simulink model "GFL_inverter"  (R2025a)
settings: Solver=ode4  StartTime=0.0  StopTime=8.5  FixedStep=1e-6  RelTol=1e-3
values from neighbouring files (symbols this model uses):
  An1 = amp1*funn    [dq_saopin_for_GFL_inverter.m]
  An2 = 0    [dq_saopin_for_GFL_inverter.m]
  An3 = 0    [dq_saopin_for_GFL_inverter.m]
  An4 = 0    [dq_saopin_for_GFL_inverter.m]
  An5 = 0    [dq_saopin_for_GFL_inverter.m]
  Ap1 = amp1*funp    [dq_saopin_for_GFL_inverter.m]
  Ap2 = 0    [dq_saopin_for_GFL_inverter.m]
  Ap3 = 0    [dq_saopin_for_GFL_inverter.m]
  Ap4 = 0    [dq_saopin_for_GFL_inverter.m]
  Ap5 = 0    [dq_saopin_for_GFL_inverter.m]
  hp1 = f    [dq_saopin_for_GFL_inverter.m]
  hp2 = f    [dq_saopin_for_GFL_inverter.m]
  hp3 = f    [dq_saopin_for_GFL_inverter.m]
  hp4 = f    [dq_saopin_for_GFL_inverter.m]
  hp5 = f    [dq_saopin_for_GFL_inverter.m]
  t_inj = 7.5    [dq_saopin_for_GFL_inverter.m]
  Ts = 5e-6    (= 5e-06)    [dq_saopin_for_GFL_inverter.m]
undefined symbols (not defined in the file or in its folder): DiscIntNeverNeededParam, level
libraries: powerlib_extras x37, spsControlledVoltageSourceLib x18, spsThreePhaseVIMeasurementLib x7, slpidlib x4, simulink_extras x4, spsabctodq0Lib x3, spsSeriesRLCBranchLib x2, spsUniversalBridgeLib x2, spsMultimeterLib x2, spsThreePhaseProgrammableVoltageSourceLib x1, spsGroundLib x1, spsIGBTDiodeLib x1
(part 1 of 2)
settings Model: SimulationMode=accelerator  Creator=18829  LastModifiedBy=wz
settings SolverCC: AlgebraicLoopSolver=TrustRegion
settings DataIOCC: ReturnWorkspaceOutputs=off
settings OptimizationCC: ReuseModelBlockBuffer=off
settings DebuggingCC: UnconnectedInputMsg=warning  UnconnectedOutputMsg=warning  UnconnectedLineMsg=warning  ArithmeticOperatorsInVariantConditions=warning
settings ModelReferenceCC: EnableRefExpFcnMdlSchedulingChecks=on
settings SFSimCC: SimUseLocalCustomCode=off  CustomCodeUndefinedFunction=UseInterfaceOnly
settings RTWCC: RTWUseLocalCustomCode=off  GPUComputeCapability=3.5
settings CodeAppCC: StateflowObjectComments=on
settings SimscapeCC: SimscapeNormalizeSystem=off

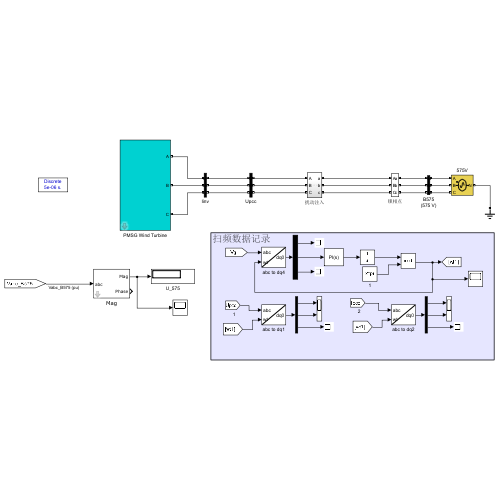
[thumbnail: Simulink's stored preview of the top-level diagram]
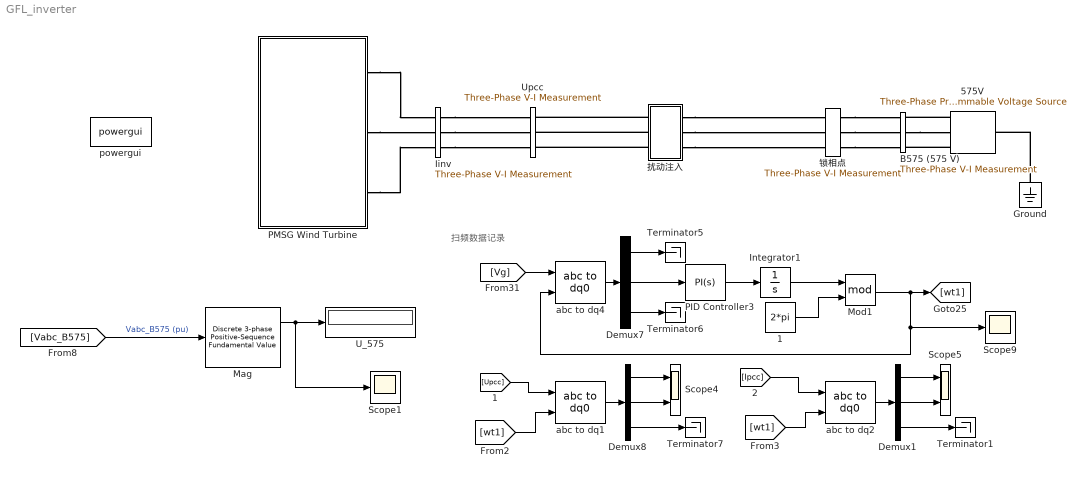
== system GFL_inverter ==
  note: 扫频数据记录
  1 : Constant  Value=2*pi
  575V : spsThreePhaseProgrammableVoltageSourceLib/Three-Phase Programmable Voltage Source  PositiveSequence=[575 0 60]  VariationEntity=Amplitude  VariationType=Table of time-amplitude pairs  VariationTypeAlt=Step  VariationStep=-0.2  VariationRate=10  VariationMagnitude=0.3  VariationFrequency=2  VariationTiming=[0.05 0.05+5/60]  VariationPhaseA=off  Amplitudes=[1 0.1 1]  TimeValues=[0 20 21]  HarmonicGeneration=off  HarmonicA=[1 -0.1 0 2]  HarmonicB=[2 0.15 35 2]*0  Timing="[0.1  2]"  BusType=swing  Pref=0  Qref=0  Qmin=-inf  Qmax=inf
  B575 (575 V) : spsThreePhaseVIMeasurementLib/Three-Phase V-I Measurement  VoltageMeasurement=phase-to-ground  SetLabelV=on  LabelV=Vabc_B575  Vpu=on  VpuLL=off  CurrentMeasurement=yes  SetLabelI=on  LabelI=Iabc_B575  Ipu=on  Pbase=1.5e6  Vbase=575  OutputType=Complex  PhasorSimulation=off  PSBequivalent=0
  Demux1 : Demux  Outputs=3
  Demux7 : Demux  Outputs=3
  Demux8 : Demux  Outputs=3
  Ground : spsGroundLib/Ground  LConnTagsString=a
  Iinv : spsThreePhaseVIMeasurementLib/Three-Phase V-I Measurement  VoltageMeasurement=no  SetLabelV=off  LabelV=Uinv  Vpu=off  VpuLL=off  CurrentMeasurement=no  SetLabelI=off  LabelI=Iinv  Ipu=off  Pbase=100e6  Vbase=500e3  OutputType=Complex  PhasorSimulation=off  PSBequivalent=0
  Integrator1 : Integrator
  Mag : powerlib_extras/Discrete Measurements/Discrete 3-phase Positive-Sequence Fundamental Value  Freq=60  Par_Init=[0 0]  Ts=Ts
  Mod1 : Math  Operator=mod  SignedPower=on
  PID Controller3 : slpidlib/PID Controller  Controller=PI  Form=Parallel  TimeDomain=Continuous-time  UseExternalTs=off  SampleTime=-1  IntegratorMethod=Forward Euler  FilterMethod=Forward Euler  ControllerParametersSource=internal  P=0.6935  I=74.885  UseKiTs=off  D=0  UseExternalDerivativeSource=off  N=100  UseFilter=on  TunerSelectOption=Transfer Function Based (PID Tuner App)  InitialConditionSource=internal  InitialConditionForIntegrator=100*pi  InitialConditionForFilter=0  DifferentiatorICPrevScaledInput=0  ExternalReset=none  TrackingMode=off  Kt=1  LimitOutput=off  SatLimitsSource=internal  UpperSaturationLimit=inf  LowerSaturationLimit=-inf  LinearizeAsGain=on  AntiWindupMode=none  Kb=1  LimitIntegrator=off  UpperIntegratorSaturationLimit=inf  LowerIntegratorSaturationLimit=-inf  POutMin=[]  POutMax=[]  IOutMin=[]  IOutMax=[]  DOutMin=[]  DOutMax=[]  NOutMin=[]  NOutMax=[]  SumOutMin=[]  SumOutMax=[]  SaturationOutMin=[]  SaturationOutMax=[]  PParamMin=[]  PParamMax=[]  IParamMin=[]  IParamMax=[]  DParamMin=[]  DParamMax=[]  NParamMin=[]  NParamMax=[]  KbParamMin=[]  KbParamMax=[]  KtParamMin=[]  KtParamMax=[]  KbOutMin=[]  KbOutMax=[]  KtOutMin=[]  KtOutMax=[]  IntegratorOutMin=[]  IntegratorOutMax=[]  FilterOutMin=[]  FilterOutMax=[]  SumI1OutMin=[]  SumI1OutMax=[]  SumI2OutMin=[]  SumI2OutMax=[]  SumI3OutMin=[]  SumI3OutMax=[]  SumI4OutMin=[]  SumI4OutMax=[]  SumDOutMin=[]  SumDOutMax=[]  DifferentiatorOutMin=[]  DifferentiatorOutMax=[]  FilterDiffOutCoefMin=[]  FilterDiffOutCoefMax=[]  ReciprocalOutMin=[]  ReciprocalOutMax=[]  SumDenOutMin=[]  SumDenOutMax=[]  SumNumOutMin=[]  SumNumOutMax=[]  DivideOutMin=[]  DivideOutMax=[]  UdiffTsProdOutMin=[]  UdiffTsProdOutMax=[]  NTsProdOutMin=[]  NTsProdOutMax=[]  UintegralTsProdOutMin=[]  UintegralTsProdOutMax=[]  UngainTsProdOutMin=[]  UngainTsProdOutMax=[]  ClampingZeroOutDataTypeStr=Inherit: Inherit via back propagation  ClampingZeroOutMin=[]  ClampingZeroOutMax=[]  FilterDenConstantOutDataTypeStr=Inherit: Inherit via back propagation  FilterDenConstantOutMin=[]  FilterDenConstantOutMax=[]  PCopyOutDataTypeStr=Inherit: Inherit via back propagation  PCopyOutMin=[]  PCopyOutMax=[]  NCopyOutDataTypeStr=Inherit: Inherit via back propagation  NCopyOutMin=[]  NCopyOutMax=[]  IntegratorContinuousStateAttributes=''  IntegratorStateMustResolveToSignalObject=off  IntegratorRTWStateStorageClass=Auto  FilterContinuousStateAttributes=''  FilterStateMustResolveToSignalObject=off  FilterRTWStateStorageClass=Auto  ParallelPVariant=InternalParameters  IdealPVariant=Disabled  IVariant=InternalParameters  DVariant=Disabled  IntegratorVariant=Continuous  SatVariant=Disabled  AWVariant=Passthrough  PCopyVariant=Disabled  TRVariant=Disabled  FdbkBlocksVariant=Forward  IdealPFdbkVariant=Disabled  SatFdbkVariant=Disabled  DerivativeFilterVariant=Disabled  NVariant=Disabled  NCopyVariant=Disabled_SignalSpec  FilterICVariant=Disabled  IntegratorICVariant=InternalICs  ExternalResetVariant=Disabled  TRSumVariant=Passthrough  SumFdbkVariant=Disabled  SumVariant=Sum_PI  TsampFilterVariant=InternalTs  TsampNgainVariant=Passthrough  TsampIntegralVariant=Disabled_SignalSpec  ExternalSaturationOutDataTypeStr=Inherit: Same as second input  DerivativeSourceVariant=Disabled  PreIntVariant=InternalPreInt
  PMSG Wind Turbine : Subsystem  mask{Vnom=575, Pnom=1.5e6, Fnom=60, RL_grid=[0.003 0.3], Vdc_nom=1150, Np=48, Fb_time_const=0.005}
      mask prompts: Vnom "Rated L-L Voltage(V)"; Pnom "Rated Power(VA)"; Fnom "Rated Frequency(Hz)"; RL_grid "Grid-side coupling impedance(p.u.)"; Vdc_nom "DC capacitor voltage(V)"; Np "Number of pole pairs"; Fb_time_const "Feed back time constant(s)"
      mask init:
      | R_RL=RL_grid(1);
      | L_RL=RL_grid(2);
  Scope1 : Scope
      settings: TimeSpan=100  ActiveDisplayYMinimum=-1  ActiveDisplayYMaximum=1  DataLoggingDecimation=200  DataLoggingVariableName=u575_Agg  DataLoggingSaveFormat=Array
  Scope4 : Scope  NumInputPorts=2
      settings: ActiveDisplayYMinimum=-49.63931  ActiveDisplayYMaximum=396.11433  DataLoggingVariableName=vdq
  Scope5 : Scope  NumInputPorts=2
      settings: ActiveDisplayYMinimum=171.67533  ActiveDisplayYMaximum=469.66107  DataLoggingVariableName=idq
  Scope9 : Scope
      settings: ActiveDisplayYMinimum=-0.78538  ActiveDisplayYMaximum=7.06841
  Terminator{1,5..7} (4 alike) : Terminator
  U_575 : Display
      settings: Decimation=10000
  Upcc : spsThreePhaseVIMeasurementLib/Three-Phase V-I Measurement  VoltageMeasurement=phase-to-ground  SetLabelV=on  LabelV=Upcc  Vpu=off  VpuLL=off  CurrentMeasurement=yes  SetLabelI=on  LabelI=Ipcc  Ipu=off  Pbase=100e6  Vbase=500e3  OutputType=Complex  PhasorSimulation=off  PSBequivalent=0
  abc to dq1 : spsabctodq0Lib/abc to dq0  Alignment=90 degrees behind phase A axis
  abc to dq2 : spsabctodq0Lib/abc to dq0  Alignment=90 degrees behind phase A axis
  abc to dq4 : spsabctodq0Lib/abc to dq0  Alignment=90 degrees behind phase A axis
  powergui : spspowerguiLib/powergui  Priority=1  SimulationMode=Discrete  SampleTime=5e-6  frequency=60  Iterations=50  frequencyindice=0  Pbase=100e6  ErrMax=1e-4  UnitsV=kV  UnitsW=MW  buscounter=0  FunctionMessages=off  echomessages=off  EnableUseOfTLC=off  CurrentSourceSwitches=off  DisableSnubberDevices=off  DisableRonSwitches=off  DisableVfSwitches=off  DisplayEquations=off  AutomaticDiscreteSolvers=off  SolverType=Tustin  Interpol=off  ExternalGateDelay=off  methode=off  Ts=0  x0status=blocks  SPID=off  SwTol=0  HookPort=off  NonlinearTolerance=1e-4  nMaxIteration=100  ContinueOnMaxIteration=off  RestoreLinks=warning  ResistiveCurrentMeasurement=off  Frange=[0:2:500]  Ylog=off  Xlog=on  ShowGrid=off  save=off  variable=ZData  structure=ScopeData1  ZoomFFT=off  StartTime=1.5  cycles=10  DisplayStyle=2  fundamental=50  FreqAxis=off  MaxFrequency=600  frequencyindicesteady=1  RmsSteady=1  display=off
  扰动注入 : Subsystem
  锁相点 : spsThreePhaseVIMeasurementLib/Three-Phase V-I Measurement  VoltageMeasurement=phase-to-ground  SetLabelV=on  LabelV=Vg  Vpu=off  VpuLL=off  CurrentMeasurement=no  SetLabelI=off  LabelI=Iabc  Ipu=off  Pbase=100e6  Vbase=500e3  OutputType=Complex  PhasorSimulation=off  PSBequivalent=0
  wires:
  1/1 -> Mod1/2
  PID Controller3/1 -> Integrator1/1
  Integrator1/1 -> Mod1/1
  Demux7/1 -> Terminator5/1
  Demux7/2 -> PID Controller3/1
  Demux7/3 -> Terminator6/1
  abc to dq4/1 -> Demux7/1
  [Vg] -> abc to dq4/1
  Mod1/1 -> [wt1], Scope9/1, abc to dq4/2
  [Upcc] -> abc to dq1/1
  [wt1] -> abc to dq1/2
  abc to dq1/1 -> Demux8/1
  Demux8/3 -> Terminator7/1
  Demux8/1 -> Scope4/1
  Demux8/2 -> Scope4/2
  Demux1/2 -> Scope5/2
  Demux1/1 -> Scope5/1
  Demux1/3 -> Terminator1/1
  abc to dq2/1 -> Demux1/1
  [wt1] -> abc to dq2/2
  [Ipcc] -> abc to dq2/1
  Mag/1 -> U_575/1, Scope1/1
  [Vabc_B575] -> Mag/1  "Vabc_B575 (pu)"
  connections:
  扰动注入/LConn1 -- Upcc/RConn1
  扰动注入/RConn1 -- 锁相点/LConn1
  扰动注入/LConn2 -- Upcc/RConn2
  扰动注入/RConn2 -- 锁相点/LConn2
  扰动注入/LConn3 -- Upcc/RConn3
  扰动注入/RConn3 -- 锁相点/LConn3
  B575 (575 V)/LConn2 -- 575V/RConn2
  Ground/LConn1 -- 575V/LConn1
  575V/RConn3 -- B575 (575 V)/LConn3
  575V/RConn1 -- B575 (575 V)/LConn1
  锁相点/RConn1 -- B575 (575 V)/RConn1
  锁相点/RConn2 -- B575 (575 V)/RConn2
  锁相点/RConn3 -- B575 (575 V)/RConn3
  PMSG Wind Turbine/RConn2 -- Iinv/LConn2
  PMSG Wind Turbine/RConn1 -- Iinv/LConn1
  PMSG Wind Turbine/RConn3 -- Iinv/LConn3
  Iinv/RConn1 -- Upcc/LConn1
  Iinv/RConn2 -- Upcc/LConn2
  Iinv/RConn3 -- Upcc/LConn3

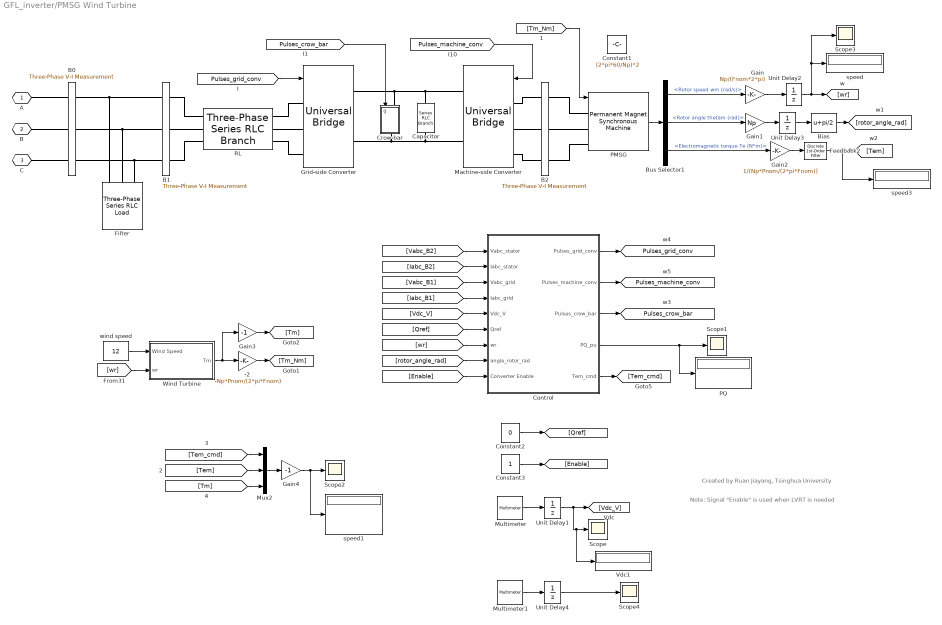
== system GFL_inverter/PMSG Wind Turbine ==
  note: Created by Ruan Jiayang, Tsinghua University
  note: Note: Signal "Enable" is used when LVRT is needed
  -2 : Gain  Gain=-Np*Pnom/(2*pi*Fnom)
  B0 : spsThreePhaseVIMeasurementLib/Three-Phase V-I Measurement  VoltageMeasurement=phase-to-ground  SetLabelV=on  LabelV=Vabc_B0  Vpu=on  VpuLL=off  CurrentMeasurement=yes  SetLabelI=on  LabelI=Iabc_B0  Ipu=on  Pbase=Pnom  Vbase=Vnom  OutputType=Complex  PhasorSimulation=off  PSBequivalent=0
  B1 : spsThreePhaseVIMeasurementLib/Three-Phase V-I Measurement  VoltageMeasurement=phase-to-ground  SetLabelV=on  LabelV=Vabc_B1  Vpu=on  VpuLL=off  CurrentMeasurement=yes  SetLabelI=on  LabelI=Iabc_B1  Ipu=on  Pbase=Pnom  Vbase=Vnom  OutputType=Complex  PhasorSimulation=off  PSBequivalent=0
  B2 : spsThreePhaseVIMeasurementLib/Three-Phase V-I Measurement  VoltageMeasurement=phase-to-ground  SetLabelV=on  LabelV=Vabc_B2  Vpu=on  VpuLL=off  CurrentMeasurement=yes  SetLabelI=on  LabelI=Iabc_B2  Ipu=on  Pbase=Pnom  Vbase=Vnom  OutputType=Complex  PhasorSimulation=off  PSBequivalent=0
  Bias : Bias  Bias=pi/2  SaturateOnIntegerOverflow=off
  Bus Selector1 : BusSelector  OutputSignals=Rotor speed wm (rad/s),Rotor angle thetam (rad),Electromagnetic torque Te (N*m)
  Capacitor : spsSeriesRLCBranchLib/Series RLC Branch  LConnTagsString=__new0  RConnTagsString=__new0  BranchType=C  Resistance=1e-5  Inductance=1e-3  SetiL0=off  InitialCurrent=0  Capacitance=10000e-6  Setx0=on  InitialVoltage=Vdc_nom  Measurements=Branch voltage
  Constant1 : Constant  Value=(2*pi*60/Np)*2  SampleTime=Ts
  Constant2 : Constant  Value=0  SampleTime=Ts
  Constant3 : Constant  SampleTime=Ts
  Control : Subsystem
  Crow-bar : Subsystem
  Feedback2 : powerlib_extras/Discrete  Control Blocks/Discrete 1st-Order Filter  FilterType=Lowpass  Tc=0.3  Ts=Ts  Initialize=on  Vac_Init=[0 -25 60]  Vdc_Init=0  PlotResponse=off  param1=[1 500 0.1]
  Filter : spsThreePhaseSeriesRLCLoadLib/Three-Phase Series RLC Load  LConnTagsString=A|B|C  Configuration=Y (grounded)  NominalVoltage=Vnom  Vabc=[1e3 1e3 1e3]  Vabcp=[1e3 1e3 1e3]  NominalFrequency=Pnom  UnbalancedPower=off  ActivePower=0.005e6  InductivePower=0  CapacitivePower=0.04e6  Pabc=[10e3 9e3 11e3]  QLabc=[100 90 110]  QCabc=[100 90 110]  Pabcp=[10e3 9e3 11e3]  QLabcp=[100 90 110]  QCabcp=[100 90 110]  Measurements=None  LoadType=constant Z
  Gain : Gain  Gain=Np/(Fnom*2*pi)
  Gain1 : Gain  Gain=Np
  Gain2 : Gain  Gain=1/(Np*Pnom/(2*pi*Fnom))
  Gain3 : Gain  Gain=-1
  Gain4 : Gain  Gain=-1
  Grid-side Converter : spsUniversalBridgeLib/Universal Bridge  Arms=3  SnubberResistance=1e5  SnubberCapacitance=inf  Device=IGBT / Diodes  Ron=1e-5  Lon=0  ForwardVoltages="[  0  0  ]"  ForwardVoltage=0  GTOparameters=[ 10e-6 , 20e-6 ]  IGBTparameters=[0 , 0]  Measurements=None  Measurements_2=None  converterType=Rectifier
  Machine-side Converter : spsUniversalBridgeLib/Universal Bridge  Arms=3  SnubberResistance=1e5  SnubberCapacitance=inf  Device=IGBT / Diodes  Ron=1e-5  Lon=0  ForwardVoltages="[  0  0  ]"  ForwardVoltage=0  GTOparameters=[ 10e-6 , 20e-6 ]  IGBTparameters=[0 , 0]  Measurements=None  Measurements_2=None  converterType=Rectifier
  Multimeter : spsMultimeterLib/Multimeter  L=2  sel=1  yselected={}  Gain=1  OutputType=Complex  PlotAtSimulationStop=off  PhasorSimulation=off
  Multimeter1 : spsMultimeterLib/Multimeter  L=2  sel=2  yselected={}  Gain=1  OutputType=Complex  PlotAtSimulationStop=off  PhasorSimulation=off
  Mux2 : Mux  Inputs=3
  PMSG : spsPermanentMagnetSynchronousMachineLib/Permanent Magnet Synchronous Machine  NbPhases=3  FluxDistribution=Sinusoidal  RotorType=Salient-pole  MechanicalLoad=Torque Tm  PresetModel=No  ShowDetailedParameters=on  MeasurementBus=off  Resistance=0.006  Inductance=8.5e-3  dqInductances="[0.3e-3  0.3e-3]"  La=0.000395  MachineConstant=Flux linkage established by magnets (V.s)  Flux=1.48  VoltageCst=12885.2307  TorqueCst=106.56  Flat=120  Mechanical=[35000 0.01 Np]  PolePairs=Np  InitialConditions=[(2*pi*Fnom/Np)*1,0, 0,0]  InitialConditions5ph=[0 0 0 0 0 0]  RefAngle=90 degrees behind phase A axis (modified Park)  IterativeDiscreteModel=Trapezoidal non iterative  TsBlock=Ts  TsPowergui=0
  PQ : Display
      settings: Decimation=10000
  RL : spsThreePhaseSeriesRLCBranchLib/Three-Phase Series RLC Branch  LConnTagsString=A|B|C  RConnTagsString=A|B|C  BranchType=RL  Resistance=R_RL*Vnom^2/Pnom  Inductance=L_RL*Vnom^2/Pnom/(2*pi*Fnom)  Capacitance=1.0  Measurements=None
  Scope{,1..4} (5 alike) : Scope
      Scope settings: DataLoggingDecimation=100
      Scope1 settings: ActiveDisplayYMinimum=-0.16459703024448283  ActiveDisplayYMaximum=1.0547130308435688  DataLoggingDecimation=100
      Scope2 settings: ActiveDisplayYMinimum=-0.1  ActiveDisplayYMaximum=0.3  DataLoggingDecimation=100  DataLoggingVariableName=ScopeData6
      Scope3 settings: DataLoggingDecimation=100  DataLoggingVariableName=ScopeData9
      Scope4 settings: TimeSpan=35  ActiveDisplayYMinimum=0  ActiveDisplayYMaximum=2000  DataLoggingDecimation=100  DataLoggingVariableName=ScopeData5
  Unit Delay{1..4} (4 alike) : UnitDelay  SampleTime=Ts
  Vdc1 : Display
      settings: Decimation=10000
  Wind Turbine : Subsystem
  speed : Display
      settings: Decimation=10000
  speed1 : Display
      settings: Decimation=10000
  speed3 : Display
      settings: Decimation=1000
  wind speed : Constant  Value=12
  A : PMIOPort  Tag=PMCPort  Side=Right
  B : PMIOPort  Tag=PMCPort  Port=2  Side=Right
  C : PMIOPort  Tag=PMCPort  Port=3  Side=Right
  tag scope: Pulses_crow_bar=global, Pulses_grid_conv=global, Pulses_machine_conv=global
  wires:
  Unit Delay1/1 -> [Vdc_V], Scope/1, Vdc1/1
  PMSG/1 -> Bus Selector1/1
  Bus Selector1/1 -> Gain/1  "<Rotor speed wm (rad/s)>"
  Gain/1 -> Unit Delay2/1
  Gain1/1 -> Unit Delay3/1
  Bus Selector1/2 -> Gain1/1  "<Rotor angle thetam (rad)>"
  Unit Delay2/1 -> [wr], speed/1, Scope3/1
  [Qref] -> Control/6(Qref)
  [Vdc_V] -> Control/5(Vdc_V)
  [Iabc_B1] -> Control/4(Iabc_grid)
  [Vabc_B1] -> Control/3(Vabc_grid)
  [Vabc_B2] -> Control/1(Vabc_stator)
  [Iabc_B2] -> Control/2(Iabc_stator)
  [Enable] -> Control/9(Converter Enable)
  Constant3/1 -> [Enable]
  Constant2/1 -> [Qref]
  [Pulses_grid_conv] -> Grid-side Converter/1
  [Pulses_machine_conv] -> Machine-side Converter/1
  Control/1(Pulses_grid_conv) -> [Pulses_grid_conv]
  Control/4(PQ_pu) -> Scope1/1, PQ/1
  Control/2(Pulses_machine_conv) -> [Pulses_machine_conv]
  [wr] -> Control/7(wr)
  [rotor_angle_rad] -> Control/8(angle_rotor_rad)
  Bus Selector1/3 -> Gain2/1  "<Electromagnetic torque Te (N*m)>"
  Bias/1 -> [rotor_angle_rad]
  Unit Delay3/1 -> Bias/1
  Wind Turbine/1(Tm) -> -2/1, Gain3/1
  -2/1 -> [Tm_Nm]
  [wr] -> Wind Turbine/2(wr)
  wind speed/1 -> Wind Turbine/1(Wind Speed)
  [Tm_Nm] -> PMSG/1
  Gain2/1 -> Feedback2/1
  Feedback2/1 -> [Tem], speed3/1
  Control/5(Tem_cmd) -> [Tem_cmd]
  [Tem] -> Mux2/2
  [Tem_cmd] -> Mux2/1
  [Tm] -> Mux2/3
  Mux2/1 -> Gain4/1
  Gain4/1 -> Scope2/1, speed1/1
  Gain3/1 -> [Tm]
  Multimeter/1 -> Unit Delay1/1
  Control/3(Pulses_crow_bar) -> [Pulses_crow_bar]
  Unit Delay4/1 -> Scope4/1
  Multimeter1/1 -> Unit Delay4/1
  [Pulses_crow_bar] -> Crow-bar/1(g)
  connections:
  RL/RConn1 -- Grid-side Converter/LConn1
  RL/RConn2 -- Grid-side Converter/LConn2
  RL/RConn3 -- Grid-side Converter/LConn3
  B1/LConn1 -- Filter/LConn1 -- B0/RConn1
  B1/LConn2 -- Filter/LConn2 -- B0/RConn2
  B1/LConn3 -- Filter/LConn3 -- B0/RConn3
  B1/RConn1 -- RL/LConn1
  RL/LConn2 -- B1/RConn2
  B1/RConn3 -- RL/LConn3
  B2/RConn2 -- PMSG/LConn2
  PMSG/LConn1 -- B2/RConn1
  B2/LConn1 -- Machine-side Converter/LConn1
  Machine-side Converter/LConn3 -- B2/LConn3
  B2/LConn2 -- Machine-side Converter/LConn2
  B0/LConn1 -- A/RConn1
  B/RConn1 -- B0/LConn2
  C/RConn1 -- B0/LConn3
  B2/RConn3 -- PMSG/LConn3
  Grid-side Converter/RConn1 -- Crow-bar/LConn1 -- Machine-side Converter/RConn1 -- Capacitor/LConn1
  Grid-side Converter/RConn2 -- Crow-bar/RConn1 -- Machine-side Converter/RConn2 -- Capacitor/RConn1

== system GFL_inverter/扰动注入 ==
  扰动注入1 : Subsystem  mask{Ap1=Ap1, Ap2=Ap2, Ap3=Ap3, Ap4=Ap4, Ap5=Ap5, h1=hp1, h2=hp2, h3=hp3, h4=hp4, h5=hp5}
      mask DialogControl ParameterGroupVar Prompt: 参数
  扰动注入2 : Subsystem  mask{An1=An1, An2=An2, An3=An3, An4=An4, v5=An5, h1=hp1, h2=hp2, h3=hp3, h4=hp4, h5=hp5}
      mask prompts: v5 "An5"
      mask DialogControl ParameterGroupVar Prompt: 参数
  A : PMIOPort  Side=Left
  a : PMIOPort  Port=2  Side=Right
  B : PMIOPort  Port=3  Side=Left
  b : PMIOPort  Port=4  Side=Right
  C : PMIOPort  Port=5  Side=Left
  c : PMIOPort  Port=6  Side=Right
  connections:
  扰动注入2/RConn2 -- b/RConn1
  扰动注入2/LConn1 -- 扰动注入1/RConn1
  扰动注入1/LConn2 -- B/RConn1
  扰动注入2/LConn2 -- 扰动注入1/RConn2
  扰动注入2/LConn3 -- 扰动注入1/RConn3
  扰动注入2/RConn1 -- a/RConn1
  扰动注入1/LConn1 -- A/RConn1
  扰动注入1/LConn3 -- C/RConn1
  扰动注入2/RConn3 -- c/RConn1

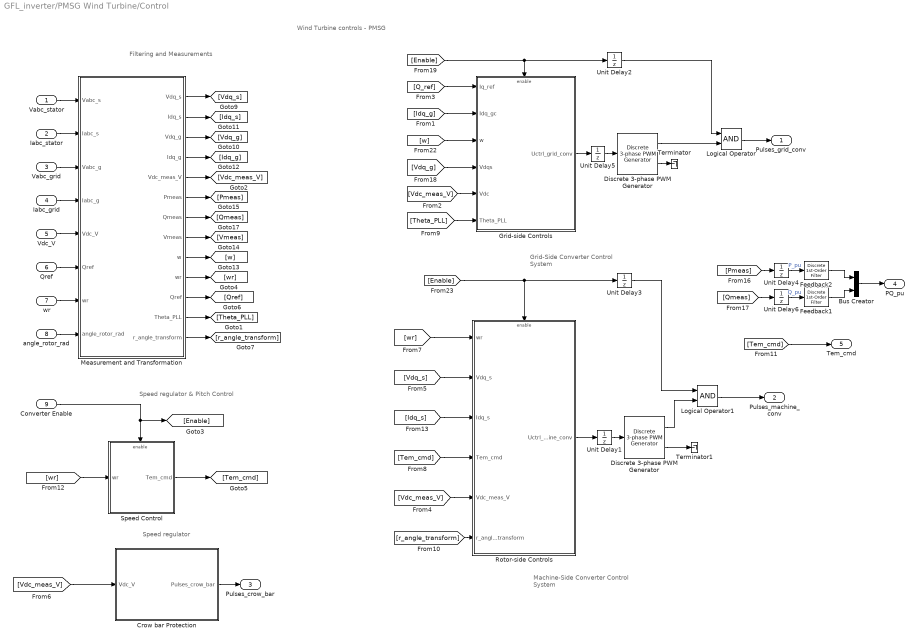
== system GFL_inverter/PMSG Wind Turbine/Control ==
  note: Wind Turbine controls - PMSG
  note: Filtering and
      | Measurements
  note: Speed regulator & Pitch Control
  note: Speed regulator
  note: Grid-Side Converter
      | Control System
  note: Machine-Side Converter
      | Control System
  Vabc_stator : Inport
  Iabc_stator : Inport  Port=2
  Vabc_grid : Inport  Port=3
  Iabc_grid : Inport  Port=4
  Vdc_V : Inport  Port=5
  Qref : Inport  Port=6
  wr : Inport  Port=7
  angle_rotor_rad : Inport  Port=8
  Converter Enable : Inport  Port=9
  Bus Creator : BusCreator  Inputs=2
  Crow bar Protection : Subsystem
  Discrete 3-phase PWM Generator : powerlib_extras/Discrete  Control Blocks/Discrete 3-phase PWM Generator  ModulatorType=2-level  ModulatorMode=Un-synchronized  nF=27  Fc=2700  ModulatingSignals=off  m=0.2  Freq=60  Phase=0  Ts=Ts
  "Discrete 3-phase PWM Generator " : powerlib_extras/Discrete  Control Blocks/Discrete 3-phase PWM Generator  ModulatorType=2-level  ModulatorMode=Un-synchronized  nF=27  Fc=1620  ModulatingSignals=off  m=0.2  Freq=60  Phase=0  Ts=Ts
  Feedback1 : powerlib_extras/Discrete  Control Blocks/Discrete 1st-Order Filter  FilterType=Lowpass  Tc=0.3  Ts=Ts  Initialize=on  Vac_Init=[0 -25 60]  Vdc_Init=0  PlotResponse=off  param1=[1 500 0.1]
  Feedback2 : powerlib_extras/Discrete  Control Blocks/Discrete 1st-Order Filter  FilterType=Lowpass  Tc=0.3  Ts=Ts  Initialize=on  Vac_Init=[0 -25 60]  Vdc_Init=0  PlotResponse=off  param1=[1 500 0.1]
  Grid-side Controls : Subsystem
  Logical Operator : Logic  AllPortsSameDT=off  OutDataTypeStr=boolean
  Logical Operator1 : Logic  AllPortsSameDT=off  OutDataTypeStr=boolean
  Measurement and Transformation : Subsystem
  Rotor-side Controls : Subsystem
  Speed Control : Subsystem
  Terminator : Terminator
  Terminator1 : Terminator
  Unit Delay{1..6} (6 alike) : UnitDelay  SampleTime=Ts
  Pulses_grid_conv : Outport
  Pulses_machine_conv : Outport  Port=2
  Pulses_crow_bar : Outport  Port=3
  PQ_pu : Outport  Port=4
  Tem_cmd : Outport  Port=5
  wires:
  [Pmeas] -> Unit Delay4/1
  [Qmeas] -> Unit Delay6/1
  wr/1 -> Measurement and Transformation/7(wr)
  Qref/1 -> Measurement and Transformation/6(Qref)
  Vdc_V/1 -> Measurement and Transformation/5(Vdc_V)
  Measurement and Transformation/11("Qref ") -> [Qref]
  Measurement and Transformation/10("wr ") -> [wr]
  Measurement and Transformation/5(Vdc_meas_V) -> [Vdc_meas_V]
  Measurement and Transformation/9(w) -> [w]
  Measurement and Transformation/6(Pmeas) -> [Pmeas]
  Measurement and Transformation/4(Idq_g) -> [Idq_g]
  Measurement and Transformation/3(Vdq_g) -> [Vdq_g]
  Measurement and Transformation/2(Idq_s) -> [Idq_s]
  angle_rotor_rad/1 -> Measurement and Transformation/8(angle_rotor_rad)
  Iabc_stator/1 -> Measurement and Transformation/2(Iabc_s)
  Iabc_grid/1 -> Measurement and Transformation/4(Iabc_g)
  Vabc_grid/1 -> Measurement and Transformation/3(Vabc_g)
  Vabc_stator/1 -> Measurement and Transformation/1(Vabc_s)
  Measurement and Transformation/7(Qmeas) -> [Qmeas]
  Measurement and Transformation/8(Vmeas) -> [Vmeas]
  Measurement and Transformation/12(Theta_PLL) -> [Theta_PLL]
  Measurement and Transformation/13(r_angle_transform) -> [r_angle_transform]
  Speed Control/1(Tem_cmd) -> [Tem_cmd]
  [wr] -> Speed Control/1(wr)
  Converter Enable/1 -> Speed Control/Enable, [Enable]
  [Tem_cmd] -> Tem_cmd/1
  Measurement and Transformation/1(Vdq_s) -> [Vdq_s]
  Grid-side Controls/1(Uctrl_grid_conv) -> Unit Delay5/1
  Discrete 3-phase PWM Generator/2 -> Terminator/1
  Unit Delay5/1 -> Discrete 3-phase PWM Generator/1
  [Vdc_meas_V] -> Grid-side Controls/5(Vdc)
  [Vdq_g] -> Grid-side Controls/4(Vdqs)
  [w] -> Grid-side Controls/3(w)
  [Idq_g] -> Grid-side Controls/2(Idq_gc)
  [Q_ref] -> Grid-side Controls/1(Iq_ref)
  [Theta_PLL] -> Grid-side Controls/6(Theta_PLL)
  [Enable] -> Grid-side Controls/Enable, Unit Delay2/1
  Logical Operator/1 -> Pulses_grid_conv/1
  Discrete 3-phase PWM Generator/1 -> Logical Operator/2
  Unit Delay2/1 -> Logical Operator/1
  "Discrete 3-phase PWM Generator "/2 -> Terminator1/1
  Unit Delay1/1 -> "Discrete 3-phase PWM Generator "/1
  [Enable] -> Unit Delay3/1, Rotor-side Controls/Enable
  Logical Operator1/1 -> Pulses_machine_conv/1
  "Discrete 3-phase PWM Generator "/1 -> Logical Operator1/2
  Unit Delay3/1 -> Logical Operator1/1
  [wr] -> Rotor-side Controls/1(wr)
  [Vdc_meas_V] -> Rotor-side Controls/5(Vdc_meas_V)
  [r_angle_transform] -> Rotor-side Controls/6(r_angle_transform)
  [Vdq_s] -> Rotor-side Controls/2(" Vdq_s")
  [Idq_s] -> Rotor-side Controls/3(Idq_s)
  Rotor-side Controls/1(Uctrl_machine_conv) -> Unit Delay1/1
  [Tem_cmd] -> Rotor-side Controls/4(Tem_cmd)
  Unit Delay4/1 -> Feedback2/1  "P_pu"
  Feedback2/1 -> Bus Creator/1
  Unit Delay6/1 -> Feedback1/1  "Q_pu"
  Feedback1/1 -> Bus Creator/2
  Crow bar Protection/1(Pulses_crow_bar) -> Pulses_crow_bar/1
  [Vdc_meas_V] -> Crow bar Protection/1(Vdc_V)
  Bus Creator/1 -> PQ_pu/1

== system GFL_inverter/PMSG Wind Turbine/Crow-bar ==
  g : Inport
  IGBT : spsIGBTDiodeLib/IGBT//Diode  Ron=1e-5  Rs=1e5  Cs=inf  Measurements=off
  R : spsSeriesRLCBranchLib/Series RLC Branch  LConnTagsString=__new0  RConnTagsString=__new0  BranchType=R  Resistance=1  Inductance=1e-3  SetiL0=off  InitialCurrent=0  Capacitance=1e-6  Setx0=off  InitialVoltage=0  Measurements=Branch current
  + : PMIOPort  Side=Left
  - : PMIOPort  Port=2  Side=Right
  wires:
  g/1 -> IGBT/1
  connections:
  R/LConn1 -- IGBT/RConn1
  +/RConn1 -- IGBT/LConn1
  -/RConn1 -- R/RConn1

== system GFL_inverter/PMSG Wind Turbine/Wind Turbine ==
  Wind Speed : Inport
  wr : Inport  Port=2
  Constant1 : Constant  Value=1.0*1.2  SampleTime=Ts
  Display : Display
      settings: Decimation=10000
  Display1 : Display
      settings: Decimation=10000
  Display2 : Display
      settings: Decimation=10000
  Scope1 : Scope
      settings: ActiveDisplayYMinimum=-1  ActiveDisplayYMaximum=2  DataLoggingDecimation=1000  DataLoggingVariableName=ScopeData2
  Scope3 : Scope
      settings: TimeSpan=18  ActiveDisplayYMinimum=1.082  ActiveDisplayYMaximum=1.102  DataLoggingDecimation=1000  DataLoggingVariableName=wr  DataLoggingSaveFormat=Array
  Turbine Rotor : Subsystem
  pitch angle controller : Subsystem
  Tm : Outport
  wires:
  Turbine Rotor/1(Tm) -> Tm/1, Display/1, Scope3/1  "Tm"
  Constant1/1 -> pitch angle controller/2(Ref)
  pitch angle controller/1(pitch) -> Scope1/1, Display1/1, Turbine Rotor/3(pitch)
  Wind Speed/1 -> Turbine Rotor/1(u), Display2/1
  wr/1 -> pitch angle controller/1(wg), Turbine Rotor/2(wr)

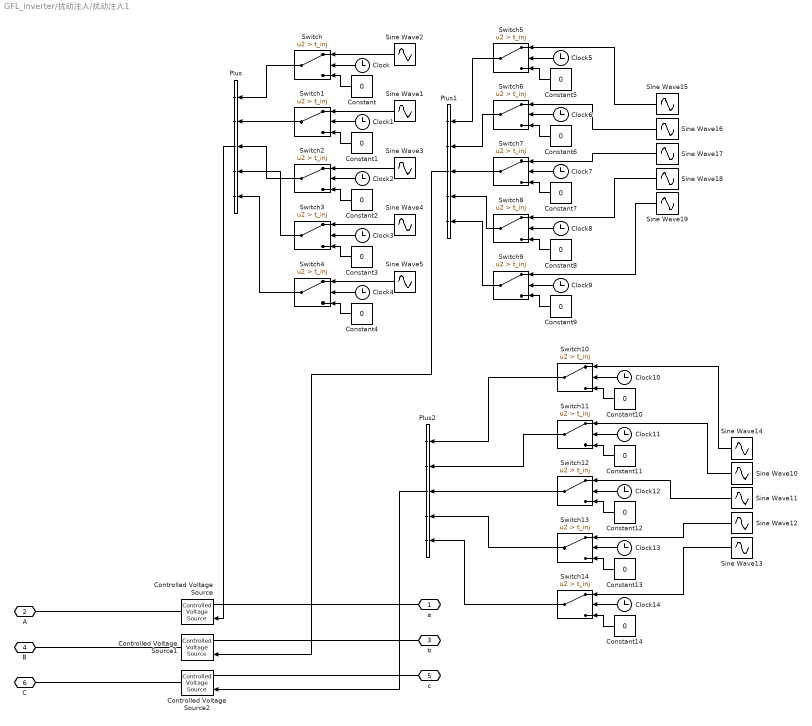
== system GFL_inverter/扰动注入/扰动注入1 ==
  Clock{,1..14} (15 alike) : Clock
  Constant{,1..14} (15 alike) : Constant  Value=0
  Controlled Voltage Source : spsControlledVoltageSourceLib/Controlled Voltage Source  Initialize=on  Source_Type=AC  Amplitude=0  Phase=0  Frequency=0  Measurements=None
  Controlled Voltage Source1 : spsControlledVoltageSourceLib/Controlled Voltage Source  Initialize=on  Source_Type=AC  Amplitude=0  Phase=0  Frequency=0  Measurements=None
  Controlled Voltage Source2 : spsControlledVoltageSourceLib/Controlled Voltage Source  Initialize=on  Source_Type=AC  Amplitude=0  Phase=0  Frequency=0  Measurements=None
  Plus : Sum  Inputs=+++++
  Plus1 : Sum  Inputs=+++++
  Plus2 : Sum  Inputs=+++++
  Sine Wave1 : Sin  Amplitude=Ap2  Frequency=2*pi*h2+2*pi*50  SampleTime=0
  Sine Wave10 : Sin  Amplitude=Ap2  Frequency=2*pi*h2+2*pi*50  Phase=+2*pi/3  SampleTime=0
  Sine Wave11 : Sin  Amplitude=Ap3  Frequency=2*pi*h3+2*pi*50  Phase=+2*pi/3  SampleTime=0
  Sine Wave12 : Sin  Amplitude=Ap4  Frequency=2*pi*h4+2*pi*50  Phase=+2*pi/3  SampleTime=0
  Sine Wave13 : Sin  Amplitude=Ap5  Frequency=2*pi*h5+2*pi*50  Phase=+2*pi/3  SampleTime=0
  Sine Wave14 : Sin  Amplitude=Ap1  Frequency=2*pi*h1+2*pi*50  Phase=+2*pi/3  SampleTime=0
  Sine Wave15 : Sin  Amplitude=Ap1  Frequency=2*pi*h1+2*pi*50  Phase=-2*pi/3  SampleTime=0
  Sine Wave16 : Sin  Amplitude=Ap2  Frequency=2*pi*h2+2*pi*50  Phase=-2*pi/3  SampleTime=0
  Sine Wave17 : Sin  Amplitude=Ap3  Frequency=2*pi*h3+2*pi*50  Phase=-2*pi/3  SampleTime=0
  Sine Wave18 : Sin  Amplitude=Ap4  Frequency=2*pi*h4+2*pi*50  Phase=-2*pi/3  SampleTime=0
  Sine Wave19 : Sin  Amplitude=Ap5  Frequency=2*pi*h5+2*pi*50  Phase=-2*pi/3  SampleTime=0
  Sine Wave2 : Sin  Amplitude=Ap1  Frequency=2*pi*h1+2*pi*50  SampleTime=0
  Sine Wave3 : Sin  Amplitude=Ap3  Frequency=2*pi*h3+2*pi*50  SampleTime=0
  Sine Wave4 : Sin  Amplitude=Ap4  Frequency=2*pi*h4+2*pi*50  SampleTime=0
  Sine Wave5 : Sin  Amplitude=Ap5  Frequency=2*pi*h5+2*pi*50  SampleTime=0
  Switch{,1..14} (15 alike) : Switch  Criteria=u2 > Threshold  Threshold=t_inj  SaturateOnIntegerOverflow=off  InputSameDT=off
  a : PMIOPort  Side=Right
  A : PMIOPort  Port=2  Side=Left
  b : PMIOPort  Port=3  Side=Right
  B : PMIOPort  Port=4  Side=Left
  c : PMIOPort  Port=5  Side=Right
  C : PMIOPort  Port=6  Side=Left
  wires:
  Plus/1 -> Controlled Voltage Source/1
  Plus1/1 -> Controlled Voltage Source1/1
  Plus2/1 -> Controlled Voltage Source2/1
  Clock/1 -> Switch/2
  Constant/1 -> Switch/3
  Constant1/1 -> Switch1/3
  Clock1/1 -> Switch1/2
  Clock3/1 -> Switch3/2
  Constant3/1 -> Switch3/3
  Constant2/1 -> Switch2/3
  Clock2/1 -> Switch2/2
  Constant4/1 -> Switch4/3
  Clock4/1 -> Switch4/2
  Sine Wave2/1 -> Switch/1
  Sine Wave1/1 -> Switch1/1
  Sine Wave3/1 -> Switch2/1
  Sine Wave4/1 -> Switch3/1
  Sine Wave5/1 -> Switch4/1
  Switch/1 -> Plus/1
  Switch1/1 -> Plus/2
  Switch2/1 -> Plus/3
  Switch3/1 -> Plus/4
  Switch4/1 -> Plus/5
  Clock9/1 -> Switch9/2
  Constant9/1 -> Switch9/3
  Clock7/1 -> Switch7/2
  Constant7/1 -> Switch7/3
  Constant8/1 -> Switch8/3
  Clock8/1 -> Switch8/2
  Clock6/1 -> Switch6/2
  Constant6/1 -> Switch6/3
  Constant5/1 -> Switch5/3
  Clock5/1 -> Switch5/2
  Sine Wave15/1 -> Switch5/1
  Sine Wave16/1 -> Switch6/1
  Sine Wave17/1 -> Switch7/1
  Sine Wave18/1 -> Switch8/1
  Sine Wave19/1 -> Switch9/1
  Switch5/1 -> Plus1/1
  Switch6/1 -> Plus1/2
  Switch7/1 -> Plus1/3
  Switch8/1 -> Plus1/4
  Switch9/1 -> Plus1/5
  Switch12/1 -> Plus2/3
  Switch13/1 -> Plus2/4
  Switch14/1 -> Plus2/5
  Switch10/1 -> Plus2/1
  Clock12/1 -> Switch12/2
  Constant14/1 -> Switch14/3
  Clock14/1 -> Switch14/2
  Clock11/1 -> Switch11/2
  Constant10/1 -> Switch10/3
  Clock13/1 -> Switch13/2
  Constant11/1 -> Switch11/3
  Switch11/1 -> Plus2/2
  Constant13/1 -> Switch13/3
  Constant12/1 -> Switch12/3
  Clock10/1 -> Switch10/2
  Sine Wave11/1 -> Switch12/1
  Sine Wave12/1 -> Switch13/1
  Sine Wave13/1 -> Switch14/1
  Sine Wave10/1 -> Switch11/1
  Sine Wave14/1 -> Switch10/1
  connections:
  Controlled Voltage Source1/LConn1 -- b/RConn1
  Controlled Voltage Source/LConn1 -- a/RConn1
  Controlled Voltage Source1/RConn1 -- B/RConn1
  Controlled Voltage Source/RConn1 -- A/RConn1
  Controlled Voltage Source2/LConn1 -- c/RConn1
  Controlled Voltage Source2/RConn1 -- C/RConn1

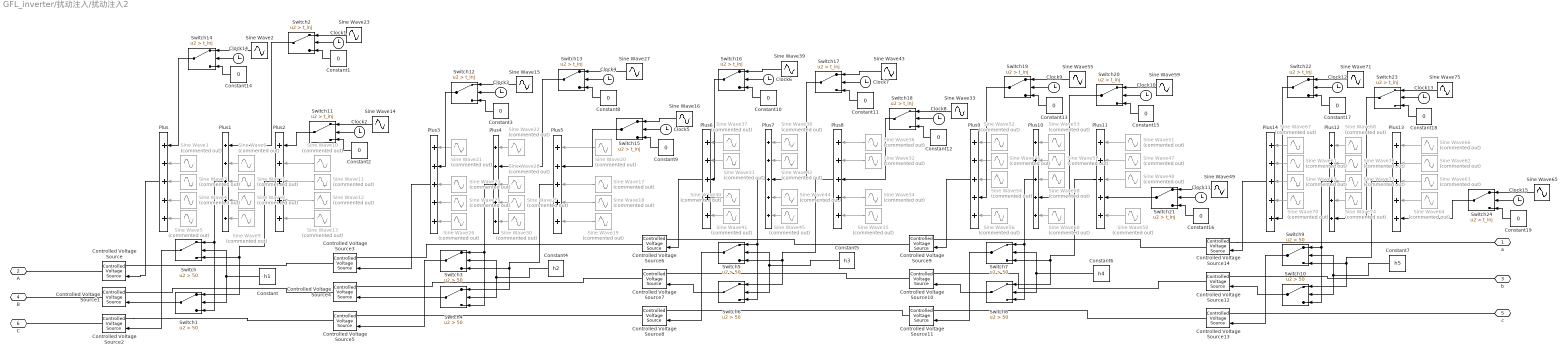
== system GFL_inverter/扰动注入/扰动注入2 ==
  Clock{1..15} (15 alike) : Clock
  Constant : Constant  Value=h1
  Constant{1..3,8..19} (15 alike) : Constant  Value=0
  Constant4 : Constant  Value=h2
  Constant5 : Constant  Value=h3
  Constant6 : Constant  Value=h4
  Constant7 : Constant  Value=h5
  Controlled Voltage Source{,1..14} (15 alike) : spsControlledVoltageSourceLib/Controlled Voltage Source  Initialize=on  Source_Type=AC  Amplitude=0  Phase=0  Frequency=0  Measurements=None
  Plus{,1..14} (15 alike) : Sum  Inputs=+++++
  Sine Wave{1,31,46,61} (4 alike) : Sin  Commented=on  Amplitude=An2  Frequency=abs(2*pi*h2-2*pi*50)  SampleTime=0
  Sine Wave{10,32,47,62} (4 alike) : Sin  Commented=on  Amplitude=An2  Frequency=abs(2*pi*h2-2*pi*50)  Phase=+2*pi/3  SampleTime=0
  Sine Wave{11,17,48,63} (4 alike) : Sin  Commented=on  Amplitude=An3  Frequency=abs(2*pi*h3-2*pi*50)  Phase=+2*pi/3  SampleTime=0
  Sine Wave12 : Sin  Commented=on  Amplitude=An4  Frequency=abs(2*pi*h4-2*pi*50)  Phase=+2*pi/3  SampleTime=0
  Sine Wave13 : Sin  Commented=on  Amplitude=An5  Frequency=abs(2*pi*h5-2*pi*50)  Phase=+2*pi/3  SampleTime=0
  Sine Wave14 : Sin  Amplitude=An1  Frequency=abs(2*pi*h1-2*pi*50)  Phase=+2*pi/3  SampleTime=0
  Sine Wave15 : Sin  Amplitude=An2  Frequency=abs(2*pi*h2-2*pi*50)  SampleTime=0
  Sine Wave16 : Sin  Amplitude=An2  Frequency=abs(2*pi*h2-2*pi*50)  Phase=+2*pi/3  SampleTime=0
  Sine Wave18 : Sin  Commented=on  Amplitude=An4  Frequency=2*pi*h4  Phase=+2*pi/3  SampleTime=0
  Sine Wave19 : Sin  Commented=on  Amplitude=An5  Frequency=2*pi*h5  Phase=+2*pi/3  SampleTime=0
  Sine Wave2 : Sin  Amplitude=An1  Frequency=abs(2*pi*h1-2*pi*50)  SampleTime=0
  Sine Wave{20,36,51,66} (4 alike) : Sin  Commented=on  Amplitude=An1  Frequency=abs(2*pi*h1-2*pi*50)  Phase=+2*pi/3  SampleTime=0
  Sine Wave{21,37,52,67} (4 alike) : Sin  Commented=on  Amplitude=An1  Frequency=abs(2*pi*h1-2*pi*50)  SampleTime=0
  Sine Wave{22,38,53,68} (4 alike) : Sin  Commented=on  Amplitude=An1  Frequency=abs(2*pi*h1-2*pi*50)  Phase=-2*pi/3  SampleTime=0
  Sine Wave23 : Sin  Amplitude=An1  Frequency=abs(2*pi*h1-2*pi*50)  Phase=-2*pi/3  SampleTime=0
  Sine Wave{3,24,54,69} (4 alike) : Sin  Commented=on  Amplitude=An3  Frequency=abs(2*pi*h3-2*pi*50)  SampleTime=0
  Sine Wave25 : Sin  Commented=on  Amplitude=An4  Frequency=2*pi*h4  SampleTime=0
  Sine Wave26 : Sin  Commented=on  Amplitude=An5  Frequency=2*pi*h5  SampleTime=0
  Sine Wave27 : Sin  Amplitude=An2  Frequency=abs(2*pi*h2-2*pi*50)  Phase=-2*pi/3  SampleTime=0
  Sine Wave{7,28,58,73} (4 alike) : Sin  Commented=on  Amplitude=An3  Frequency=abs(2*pi*h3-2*pi*50)  Phase=-2*pi/3  SampleTime=0
  Sine Wave29 : Sin  Commented=on  Amplitude=An4  Frequency=2*pi*h4  Phase=-2*pi/3  SampleTime=0
  Sine Wave30 : Sin  Commented=on  Amplitude=An5  Frequency=2*pi*h5  Phase=-2*pi/3  SampleTime=0
  Sine Wave33 : Sin  Amplitude=An3  Frequency=abs(2*pi*h3-2*pi*50)  Phase=+2*pi/3  SampleTime=0
  Sine Wave34 : Sin  Commented=on  Amplitude=An4  Frequency=2*pi*h4  Phase=+2*pi/3  SampleTime=0
  Sine Wave35 : Sin  Commented=on  Amplitude=An5  Frequency=2*pi*h5  Phase=+2*pi/3  SampleTime=0
  Sine Wave39 : Sin  Amplitude=An3  Frequency=abs(2*pi*h3-2*pi*50)  SampleTime=0
  Sine Wave4 : Sin  Commented=on  Amplitude=An4  Frequency=abs(2*pi*h4-2*pi*50)  SampleTime=0
  Sine Wave40 : Sin  Commented=on  Amplitude=An4  Frequency=2*pi*h4  SampleTime=0
  Sine Wave41 : Sin  Commented=on  Amplitude=An5  Frequency=2*pi*h5  SampleTime=0
  Sine Wave{6,42,57,72} (4 alike) : Sin  Commented=on  Amplitude=An2  Frequency=abs(2*pi*h2-2*pi*50)  Phase=-2*pi/3  SampleTime=0
  Sine Wave43 : Sin  Amplitude=An3  Frequency=abs(2*pi*h3-2*pi*50)  Phase=-2*pi/3  SampleTime=0
  Sine Wave44 : Sin  Commented=on  Amplitude=An4  Frequency=2*pi*h4  Phase=-2*pi/3  SampleTime=0
  Sine Wave45 : Sin  Commented=on  Amplitude=An5  Frequency=2*pi*h5  Phase=-2*pi/3  SampleTime=0
  Sine Wave49 : Sin  Amplitude=An4  Frequency=abs(2*pi*h4-2*pi*50)  Phase=+2*pi/3  SampleTime=0
  Sine Wave5 : Sin  Commented=on  Amplitude=An5  Frequency=abs(2*pi*h5-2*pi*50)  SampleTime=0
  Sine Wave50 : Sin  Commented=on  Amplitude=An5  Frequency=2*pi*h5  Phase=+2*pi/3  SampleTime=0
  Sine Wave55 : Sin  Amplitude=An4  Frequency=abs(2*pi*h4-2*pi*50)  SampleTime=0
  Sine Wave56 : Sin  Commented=on  Amplitude=An5  Frequency=2*pi*h5  SampleTime=0
  Sine Wave59 : Sin  Amplitude=An4  Frequency=abs(2*pi*h4-2*pi*50)  Phase=-2*pi/3  SampleTime=0
  Sine Wave60 : Sin  Commented=on  Amplitude=An5  Frequency=2*pi*h5  Phase=-2*pi/3  SampleTime=0
  Sine Wave64 : Sin  Commented=on  Amplitude=An4  Frequency=abs(2*pi*h4-2*pi*50)  Phase=+2*pi/3  SampleTime=0
  Sine Wave65 : Sin  Amplitude=An5  Frequency=abs(2*pi*h5-2*pi*50)  Phase=+2*pi/3  SampleTime=0
  Sine Wave70 : Sin  Commented=on  Amplitude=An4  Frequency=abs(2*pi*h4-2*pi*50)  SampleTime=0
  Sine Wave71 : Sin  Amplitude=An5  Frequency=abs(2*pi*h5-2*pi*50)  SampleTime=0
  Sine Wave74 : Sin  Commented=on  Amplitude=An4  Frequency=abs(2*pi*h4-2*pi*50)  Phase=-2*pi/3  SampleTime=0
  Sine Wave75 : Sin  Amplitude=An5  Frequency=abs(2*pi*h5-2*pi*50)  Phase=-2*pi/3  SampleTime=0
  Sine Wave8 : Sin  Commented=on  Amplitude=An4  Frequency=abs(2*pi*h4-2*pi*50)  Phase=-2*pi/3  SampleTime=0
  Sine Wave9 : Sin  Commented=on  Amplitude=An5  Frequency=abs(2*pi*h5-2*pi*50)  Phase=-2*pi/3  SampleTime=0
  Switch{,1,3..10} (10 alike) : Switch  Criteria=u2 > Threshold  Threshold=50  SaturateOnIntegerOverflow=off  InputSameDT=off
  Switch{2,11..24} (15 alike) : Switch  Criteria=u2 > Threshold  Threshold=t_inj  SaturateOnIntegerOverflow=off  InputSameDT=off
  a : PMIOPort  Side=Right
  A : PMIOPort  Port=2  Side=Left
  b : PMIOPort  Port=3  Side=Right
  B : PMIOPort  Port=4  Side=Left
  c : PMIOPort  Port=5  Side=Right
  C : PMIOPort  Port=6  Side=Left
  wires:
  Sine Wave13/1 -> Plus2/5
  Sine Wave12/1 -> Plus2/4
  Sine Wave11/1 -> Plus2/3
  Sine Wave10/1 -> Plus2/2
  Switch11/1 -> Plus2/1
  Sine Wave9/1 -> Plus1/5
  Sine Wave8/1 -> Plus1/4
  Sine Wave7/1 -> Plus1/3
  Switch2/1 -> Plus1/1
  Sine Wave6/1 -> Plus1/2
  Plus/1 -> Controlled Voltage Source/1
  Sine Wave5/1 -> Plus/5
  Sine Wave4/1 -> Plus/4
  Sine Wave3/1 -> Plus/3
  Sine Wave1/1 -> Plus/2
  Switch14/1 -> Plus/1
  Plus2/1 -> Switch1/1, Switch/3
  Plus1/1 -> Switch/1, Switch1/3
  Constant/1 -> Switch1/2, Switch/2
  Switch/1 -> Controlled Voltage Source2/1
  Switch1/1 -> Controlled Voltage Source1/1
  Switch4/1 -> Controlled Voltage Source4/1
  Switch3/1 -> Controlled Voltage Source5/1
  Constant4/1 -> Switch4/2, Switch3/2
  Plus4/1 -> Switch4/3, Switch3/1
  Plus5/1 -> Switch3/3, Switch4/1
  Sine Wave21/1 -> Plus3/1
  Sine Wave24/1 -> Plus3/3
  Sine Wave25/1 -> Plus3/4
  Sine Wave26/1 -> Plus3/5
  Plus3/1 -> Controlled Voltage Source3/1
  Switch13/1 -> Plus4/2
  Sine Wave22/1 -> Plus4/1
  Sine Wave28/1 -> Plus4/3
  Sine Wave29/1 -> Plus4/4
  Sine Wave30/1 -> Plus4/5
  Sine Wave20/1 -> Plus5/1
  Switch15/1 -> Plus5/2
  Sine Wave17/1 -> Plus5/3
  Sine Wave18/1 -> Plus5/4
  Sine Wave19/1 -> Plus5/5
  Sine Wave35/1 -> Plus8/5
  Sine Wave34/1 -> Plus8/4
  Sine Wave32/1 -> Plus8/2
  Sine Wave36/1 -> Plus8/1
  Sine Wave45/1 -> Plus7/5
  Sine Wave44/1 -> Plus7/4
  Switch17/1 -> Plus7/3
  Sine Wave38/1 -> Plus7/1
  Sine Wave42/1 -> Plus7/2
  Plus6/1 -> Controlled Voltage Source6/1
  Sine Wave41/1 -> Plus6/5
  Sine Wave40/1 -> Plus6/4
  Switch16/1 -> Plus6/3
  Sine Wave31/1 -> Plus6/2
  Sine Wave37/1 -> Plus6/1
  Plus8/1 -> Switch6/1, Switch5/3
  Plus7/1 -> Switch5/1, Switch6/3
  Constant5/1 -> Switch6/2, Switch5/2
  Switch5/1 -> Controlled Voltage Source8/1
  Switch6/1 -> Controlled Voltage Source7/1
  Switch8/1 -> Controlled Voltage Source10/1
  Switch7/1 -> Controlled Voltage Source11/1
  Constant6/1 -> Switch7/2, Switch8/2
  Plus10/1 -> Switch8/3, Switch7/1
  Plus11/1 -> Switch7/3, Switch8/1
  Sine Wave52/1 -> Plus9/1
  Sine Wave46/1 -> Plus9/2
  Sine Wave54/1 -> Plus9/3
  Sine Wave56/1 -> Plus9/5
  Plus9/1 -> Controlled Voltage Source9/1
  Sine Wave57/1 -> Plus10/2
  Sine Wave53/1 -> Plus10/1
  Sine Wave58/1 -> Plus10/3
  Switch20/1 -> Plus10/4
  Sine Wave60/1 -> Plus10/5
  Sine Wave51/1 -> Plus11/1
  Sine Wave47/1 -> Plus11/2
  Sine Wave48/1 -> Plus11/3
  Sine Wave50/1 -> Plus11/5
  Switch24/1 -> Plus13/5
  Sine Wave64/1 -> Plus13/4
  Sine Wave63/1 -> Plus13/3
  Sine Wave62/1 -> Plus13/2
  Sine Wave66/1 -> Plus13/1
  Switch23/1 -> Plus12/5
  Sine Wave74/1 -> Plus12/4
  Sine Wave73/1 -> Plus12/3
  Sine Wave68/1 -> Plus12/1
  Sine Wave72/1 -> Plus12/2
  Plus14/1 -> Controlled Voltage Source14/1
  Switch22/1 -> Plus14/5
  Sine Wave70/1 -> Plus14/4
  Sine Wave69/1 -> Plus14/3
  Sine Wave61/1 -> Plus14/2
  Sine Wave67/1 -> Plus14/1
  Plus13/1 -> Switch10/1, Switch9/3
  Plus12/1 -> Switch9/1, Switch10/3
  Constant7/1 -> Switch10/2, Switch9/2
  Switch9/1 -> Controlled Voltage Source13/1
  Switch10/1 -> Controlled Voltage Source12/1
  Clock14/1 -> Switch14/2
  Constant14/1 -> Switch14/3
  Sine Wave2/1 -> Switch14/1
  Sine Wave23/1 -> Switch2/1
  Constant1/1 -> Switch2/3
  Clock1/1 -> Switch2/2
  Clock2/1 -> Switch11/2
  Constant2/1 -> Switch11/3
  Sine Wave14/1 -> Switch11/1
  Sine Wave15/1 -> Switch12/1
  Clock3/1 -> Switch12/2
  Constant3/1 -> Switch12/3
  Switch12/1 -> Plus3/2
  Constant8/1 -> Switch13/3
  Clock4/1 -> Switch13/2
  Sine Wave27/1 -> Switch13/1
  Clock5/1 -> Switch15/2
  Constant9/1 -> Switch15/3
  Sine Wave16/1 -> Switch15/1
  Sine Wave39/1 -> Switch16/1
  Constant10/1 -> Switch16/3
  Clock6/1 -> Switch16/2
  Clock7/1 -> Switch17/2
  Constant11/1 -> Switch17/3
  Sine Wave43/1 -> Switch17/1
  Constant12/1 -> Switch18/3
  Sine Wave33/1 -> Switch18/1
  Clock8/1 -> Switch18/2
  Switch18/1 -> Plus8/3
  Sine Wave55/1 -> Switch19/1
  Clock9/1 -> Switch19/2
  Constant13/1 -> Switch19/3
  Switch19/1 -> Plus9/4
  Clock10/1 -> Switch20/2
  Constant15/1 -> Switch20/3
  Sine Wave59/1 -> Switch20/1
  Sine Wave49/1 -> Switch21/1
  Constant16/1 -> Switch21/3
  Clock11/1 -> Switch21/2
  Switch21/1 -> Plus11/4
  Clock12/1 -> Switch22/2
  Constant17/1 -> Switch22/3
  Sine Wave71/1 -> Switch22/1
  Constant18/1 -> Switch23/3
  Clock13/1 -> Switch23/2
  Sine Wave75/1 -> Switch23/1
  Clock15/1 -> Switch24/2
  Constant19/1 -> Switch24/3
  Sine Wave65/1 -> Switch24/1
  connections:
  Controlled Voltage Source2/RConn1 -- C/RConn1
  Controlled Voltage Source/RConn1 -- A/RConn1
  Controlled Voltage Source1/RConn1 -- B/RConn1
  Controlled Voltage Source3/RConn1 -- Controlled Voltage Source/LConn1
  Controlled Voltage Source4/RConn1 -- Controlled Voltage Source1/LConn1
  Controlled Voltage Source2/LConn1 -- Controlled Voltage Source5/RConn1
  Controlled Voltage Source6/RConn1 -- Controlled Voltage Source3/LConn1
  Controlled Voltage Source7/RConn1 -- Controlled Voltage Source4/LConn1
  Controlled Voltage Source8/RConn1 -- Controlled Voltage Source5/LConn1
  Controlled Voltage Source9/RConn1 -- Controlled Voltage Source6/LConn1
  Controlled Voltage Source10/RConn1 -- Controlled Voltage Source7/LConn1
  Controlled Voltage Source11/RConn1 -- Controlled Voltage Source8/LConn1
  Controlled Voltage Source14/RConn1 -- Controlled Voltage Source9/LConn1
  Controlled Voltage Source12/RConn1 -- Controlled Voltage Source10/LConn1
  Controlled Voltage Source13/RConn1 -- Controlled Voltage Source11/LConn1
  Controlled Voltage Source14/LConn1 -- a/RConn1
  b/RConn1 -- Controlled Voltage Source12/LConn1
  c/RConn1 -- Controlled Voltage Source13/LConn1

== system GFL_inverter/PMSG Wind Turbine/Control/Crow bar Protection ==
  Vdc_V : Inport
  Relay : Relay  OnSwitchValue=1500  OffSwitchValue=1300
  Pulses_crow_bar : Outport
  wires:
  Vdc_V/1 -> Relay/1
  Relay/1 -> Pulses_crow_bar/1

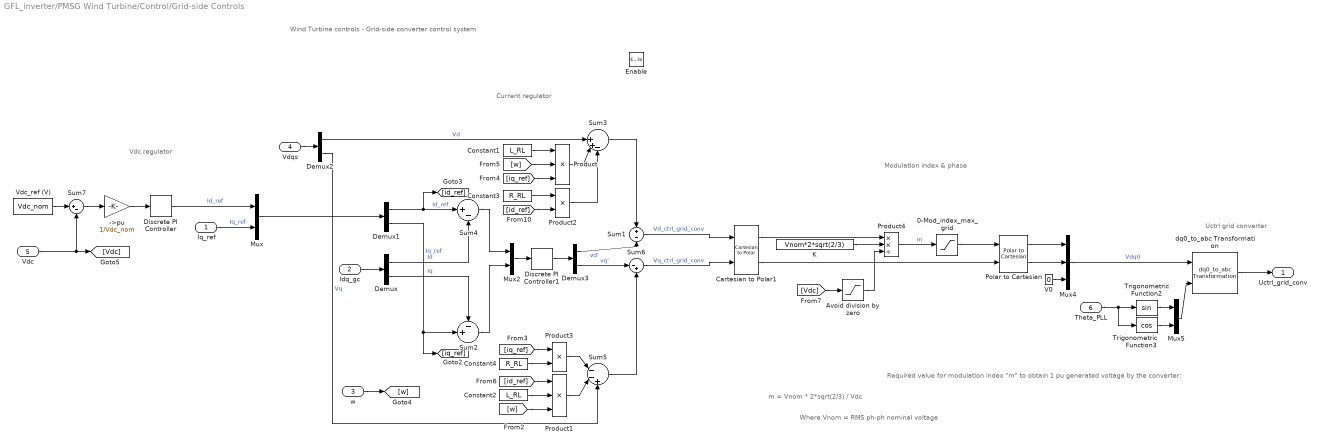
== system GFL_inverter/PMSG Wind Turbine/Control/Grid-side Controls ==
  note: Wind Turbine controls - Grid-side converter control system
  note: Where Vnom = RMS ph-ph nominal voltage
  note: m = Vnom * 2*sqrt(2/3) / Vdc
  note: Required value for modulation index "m" to obtain 1 pu generated voltage by the converter:
  note: Vdc regulator
  note: Current regulator
  note: Modulation index & phase
  note: Uctrl grid converter
  Iq_ref : Inport
  Idq_gc : Inport  Port=2
  w : Inport  Port=3
  Vdqs : Inport  Port=4
  Vdc : Inport  Port=5
  Theta_PLL : Inport  Port=6
  Enable : EnablePort
  ->pu : Gain  Gain=1/Vdc_nom
  0-Mod_index_max_grid : Saturate  UpperLimit=1.1  LowerLimit=0
  Avoid division by zero : Saturate  UpperLimit=inf  LowerLimit=1e-6
  Cartesian to Polar1 : simulink_extras/Transformations/Cartesian to Polar
  Constant1 : Constant  Value=L_RL
  Constant2 : Constant  Value=L_RL
  Constant3 : Constant  Value=R_RL
  Constant4 : Constant  Value=R_RL
  Demux{,1..3} (4 alike) : Demux  Outputs=2
      settings: DisplayOption=none
  Discrete PI Controller : powerlib_extras/Discrete  Control Blocks/Discrete PI Controller  Kp=8  Ki=400  Par_Limits=[1 -1]*1.2  Init=0  Ts=Ts
  Discrete PI Controller1 : powerlib_extras/Discrete  Control Blocks/Discrete PI Controller  Kp=0.83  Ki=5  Par_Limits=[1.0 -1.0] *1.1  Init=0  Ts=Ts
  K : Constant  Value=Vnom*2*sqrt(2/3)
  Mux : Mux  Inputs=2
  Mux2 : Mux  Inputs=2
  Mux4 : Mux  Inputs=3
  Mux5 : Mux  Inputs=2
  Polar to Cartesian : simulink_extras/Transformations/Polar to Cartesian
  Product : Product  Inputs=3  InputSameDT=on  SaturateOnIntegerOverflow=on  OutDataTypeStr=Inherit: Same as first input
  Product1 : Product  Inputs=3  InputSameDT=on  SaturateOnIntegerOverflow=on  OutDataTypeStr=Inherit: Same as first input
  Product2 : Product  InputSameDT=on  SaturateOnIntegerOverflow=on  OutDataTypeStr=Inherit: Same as first input
  Product3 : Product  InputSameDT=on  SaturateOnIntegerOverflow=on  OutDataTypeStr=Inherit: Same as first input
  Product4 : Product  Inputs=**/  InputSameDT=on  SaturateOnIntegerOverflow=on  OutDataTypeStr=Inherit: Same as first input
  Sum1 : Sum  Inputs=+-  InputSameDT=on  SaturateOnIntegerOverflow=on  OutDataTypeStr=Inherit: Same as first input
  Sum2 : Sum  Inputs=-+|  InputSameDT=on  SaturateOnIntegerOverflow=on  OutDataTypeStr=Inherit: Same as first input
  Sum3 : Sum  Inputs=||++-  InputSameDT=on  SaturateOnIntegerOverflow=on  OutDataTypeStr=Inherit: Same as first input
  Sum4 : Sum  Inputs=|+-  InputSameDT=on  SaturateOnIntegerOverflow=on  OutDataTypeStr=Inherit: Same as first input
  Sum5 : Sum  Inputs=|--+  InputSameDT=on  SaturateOnIntegerOverflow=on  OutDataTypeStr=Inherit: Same as first input
  Sum6 : Sum  Inputs=|-+  InputSameDT=on  SaturateOnIntegerOverflow=on  OutDataTypeStr=Inherit: Same as first input
  Sum7 : Sum  Inputs=|+-  InputSameDT=on  SaturateOnIntegerOverflow=on  OutDataTypeStr=Inherit: Same as first input
  Trigonometric Function2 : Trigonometry
  Trigonometric Function3 : Trigonometry  Operator=cos
  V0 : Constant  Value=0
  Vdc_ref (V) : Constant  Value=Vdc_nom
  dq0_to_abc Transformation : powerlib_extras/Measurements/dq0_to_abc Transformation
  Uctrl_grid_conv : Outport
  wires:
  Vdc_ref (V)/1 -> Sum7/1
  Iq_ref/1 -> Mux/2  "Iq_ref"
  Vdc/1 -> Sum7/2, [Vdc]
  ->pu/1 -> Discrete PI Controller/1
  Sum7/1 -> ->pu/1
  Discrete PI Controller/1 -> Mux/1  "Id_ref"
  Sum5/1 -> Sum6/2
  Sum3/1 -> Sum1/1
  Demux1/1 -> [id_ref], Sum4/1  "Id_ref"
  Demux1/2 -> Sum2/2, [iq_ref]  "Iq_ref"
  Demux3/2 -> Sum6/1  "vq'"
  Demux3/1 -> Sum1/2  "vd'"
  [id_ref] -> Product1/1
  [iq_ref] -> Product3/1
  [id_ref] -> Product2/2
  [iq_ref] -> Product/3
  [w] -> Product/2
  [w] -> Product1/3
  Sum2/1 -> Mux2/2
  Sum4/1 -> Mux2/1
  Product3/1 -> Sum5/1
  Product2/1 -> Sum3/3
  Demux2/2 -> Sum5/3  "Vq"
  Product1/1 -> Sum5/2
  Constant4/1 -> Product3/2
  Constant3/1 -> Product2/1
  Product/1 -> Sum3/2
  Demux/1 -> Sum4/2  "Id"
  Demux/2 -> Sum2/1  "Iq"
  Vdqs/1 -> Demux2/1
  Constant1/1 -> Product/1
  Demux2/1 -> Sum3/1  "Vd"
  Mux2/1 -> Discrete PI Controller1/1
  Discrete PI Controller1/1 -> Demux3/1
  Constant2/1 -> Product1/2
  w/1 -> [w]
  Idq_gc/1 -> Demux/1
  Mux/1 -> Demux1/1
  Cartesian to Polar1/2 -> Polar to Cartesian/2
  0-Mod_index_max_grid/1 -> Polar to Cartesian/1
  Cartesian to Polar1/1 -> Product4/1
  Avoid division by zero/1 -> Product4/3
  K/1 -> Product4/2
  Product4/1 -> 0-Mod_index_max_grid/1  "m"
  [Vdc] -> Avoid division by zero/1
  Mux5/1 -> dq0_to_abc Transformation/2
  Trigonometric Function2/1 -> Mux5/1
  Trigonometric Function3/1 -> Mux5/2
  V0/1 -> Mux4/3
  Polar to Cartesian/1 -> Mux4/1
  Polar to Cartesian/2 -> Mux4/2
  Mux4/1 -> dq0_to_abc Transformation/1  "Vdq0"
  Theta_PLL/1 -> Trigonometric Function3/1, Trigonometric Function2/1
  dq0_to_abc Transformation/1 -> Uctrl_grid_conv/1
  Sum1/1 -> Cartesian to Polar1/1  "Vd_ctrl_grid_conv"
  Sum6/1 -> Cartesian to Polar1/2  "Vq_ctrl_grid_conv"
